simulink model "AS_KPI"  (R2024b)
settings: Solver=VariableStepAuto  StartTime=0.0  StopTime=10.0  RelTol=1e-3
settings Model: Creator=wangjianhai  LastModifiedBy=wangjianhai
settings ConfigComp: CovBoundaryAbsTol=1.0e-5

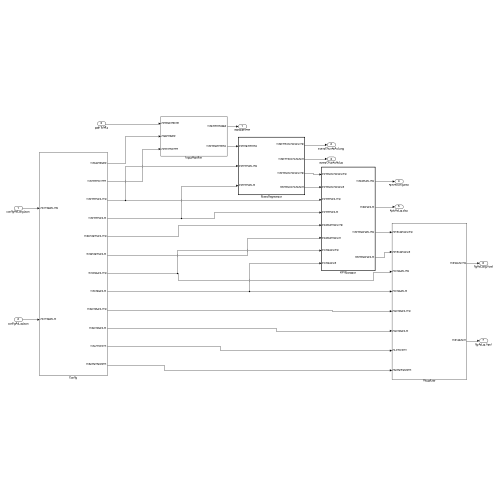
[thumbnail: Simulink's stored preview of the top-level diagram]
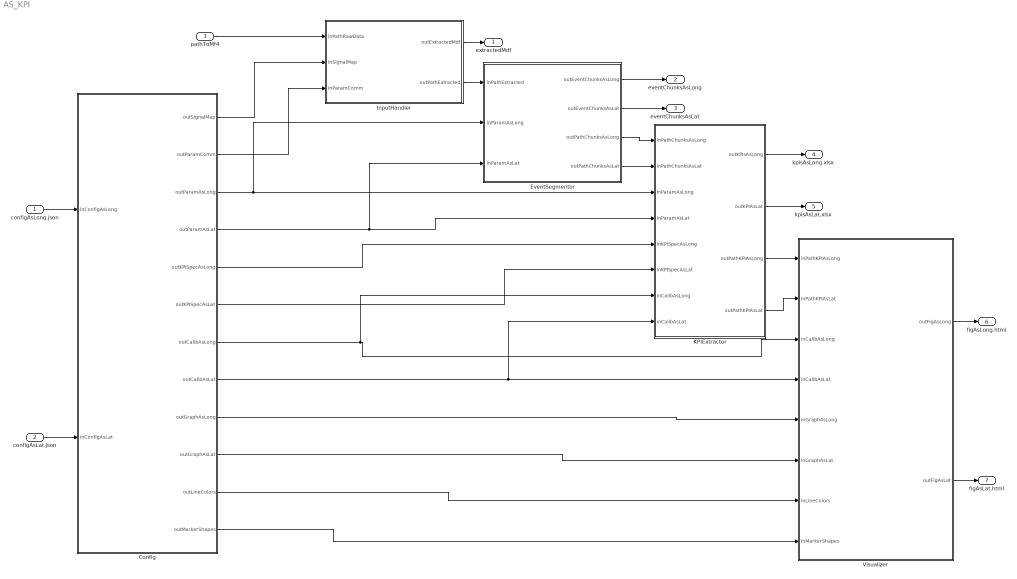
== system AS_KPI ==
  configAsLong.json : Inport
  configAsLat.json : Inport  Port=2
  pathToMf4 : Inport  Port=3
  Config : Subsystem
  EventSegmentor : Subsystem  TreatAsAtomicUnit=on
  InputHandler : Subsystem
  KPIExtractor : Subsystem  AutoFrameSizeCalculation=on
  Visualizer : Subsystem
  extractedMdf : Outport  VectorParamsAs1DForOutWhenUnconnected=off
  eventChunksAsLong : Outport  Port=2  VectorParamsAs1DForOutWhenUnconnected=off
  eventChunksAsLat : Outport  Port=3  VectorParamsAs1DForOutWhenUnconnected=off
  kpisAsLong.xlsx : Outport  Port=4  VectorParamsAs1DForOutWhenUnconnected=off
  kpisAsLat.xlsx : Outport  Port=5  VectorParamsAs1DForOutWhenUnconnected=off
  figAsLong.html : Outport  Port=6  VectorParamsAs1DForOutWhenUnconnected=off
  figAsLat.html : Outport  Port=7  VectorParamsAs1DForOutWhenUnconnected=off
  wires:
  Visualizer/2(outFigAsLat) -> figAsLat.html/1
  KPIExtractor/4(outPathKPIAsLat) -> Visualizer/2(inPathKPIAsLat)
  KPIExtractor/2(outKPIAsLat) -> kpisAsLat.xlsx/1
  KPIExtractor/1(outKPIsAsLong) -> kpisAsLong.xlsx/1
  InputHandler/2(outPathExtracted) -> EventSegmentor/1(inPathExtracted)
  Config/1(outSignalMap) -> InputHandler/2(inSignalMap)
  Config/11(outLineColors) -> Visualizer/7(inLineColors)
  Config/9(outGraphAsLong) -> Visualizer/5(inGraphAsLong)
  Config/10(outGraphAsLat) -> Visualizer/6(inGraphAsLat)
  EventSegmentor/3(outPathChunksAsLong) -> KPIExtractor/1(inPathChunksAsLong)
  Visualizer/1(outFigAsLong) -> figAsLong.html/1
  Config/7(outCalibAsLong) -> KPIExtractor/7(inCalibAsLong), Visualizer/3(inCalibAsLong)
  KPIExtractor/3(outPathKPIAsLong) -> Visualizer/1(inPathKPIAsLong)
  EventSegmentor/1(outEventChunksAsLong) -> eventChunksAsLong/1
  InputHandler/1(outExtractedMdf) -> extractedMdf/1
  Config/5(outKPISpecAsLong) -> KPIExtractor/5(inKPISpecAsLong)
  Config/4(outParamAsLat) -> EventSegmentor/3(inParamAsLat), KPIExtractor/4(inParamAsLat)
  Config/3(outParamAsLong) -> EventSegmentor/2(inParamAsLong), KPIExtractor/3(inParamAsLong)
  Config/12(outMarkerShapes) -> Visualizer/8(inMarkerShapes)
  Config/2(outParamComm) -> InputHandler/3(inParamComm)
  EventSegmentor/4(outPathChunksAsLat) -> KPIExtractor/2(inPathChunksAsLat)
  Config/8(outCalibAsLat) -> Visualizer/4(inCalibAsLat), KPIExtractor/8(inCalibAsLat)
  pathToMf4/1 -> InputHandler/1(inPathRawData)
  EventSegmentor/2(outEventChunksAsLat) -> eventChunksAsLat/1
  Config/6(outKPISpecAsLat) -> KPIExtractor/6(inKPISpecAsLat)
  configAsLat.json/1 -> Config/2(inConfigAsLat)
  configAsLong.json/1 -> Config/1(inConfigAsLong)

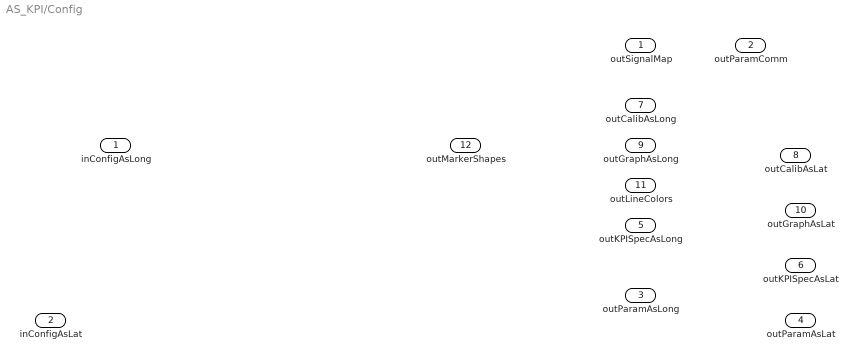
== system AS_KPI/Config ==
  inConfigAsLong : Inport
  inConfigAsLat : Inport  Port=2
  outSignalMap : Outport
  outParamComm : Outport  Port=2
  outParamAsLong : Outport  Port=3
  outParamAsLat : Outport  Port=4
  outKPISpecAsLong : Outport  Port=5
  outKPISpecAsLat : Outport  Port=6
  outCalibAsLong : Outport  Port=7
  outCalibAsLat : Outport  Port=8
  outGraphAsLong : Outport  Port=9
  outGraphAsLat : Outport  Port=10
  outLineColors : Outport  Port=11
  outMarkerShapes : Outport  Port=12

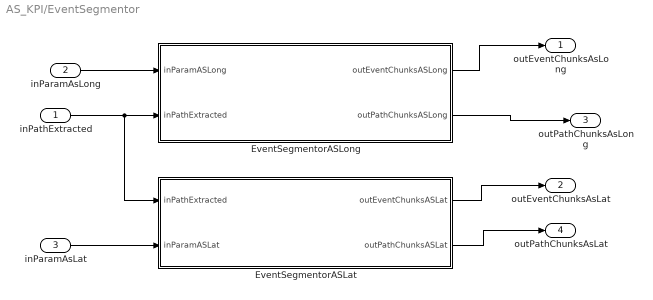
== system AS_KPI/EventSegmentor ==
  inPathExtracted : Inport
  inParamAsLong : Inport  Port=2
  inParamAsLat : Inport  Port=3
  EventSegmentorASLat : Subsystem  TreatAsAtomicUnit=on
  EventSegmentorASLong : Subsystem  TreatAsAtomicUnit=on
  outEventChunksAsLong : Outport
  outEventChunksAsLat : Outport  Port=2
  outPathChunksAsLong : Outport  Port=3
  outPathChunksAsLat : Outport  Port=4
  wires:
  inPathExtracted/1 -> EventSegmentorASLat/1(inPathExtracted), EventSegmentorASLong/2(inPathExtracted)
  inParamAsLong/1 -> EventSegmentorASLong/1(inParamASLong)
  inParamAsLat/1 -> EventSegmentorASLat/2(inParamASLat)
  EventSegmentorASLong/1(outEventChunksASLong) -> outEventChunksAsLong/1
  EventSegmentorASLong/2(outPathChunksASLong) -> outPathChunksAsLong/1
  EventSegmentorASLat/1(outEventChunksASLat) -> outEventChunksAsLat/1
  EventSegmentorASLat/2(outPathChunksASLat) -> outPathChunksAsLat/1

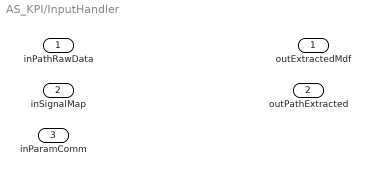
== system AS_KPI/InputHandler ==
  inPathRawData : Inport
  inSignalMap : Inport  Port=2
  inParamComm : Inport  Port=3
  outExtractedMdf : Outport
  outPathExtracted : Outport  Port=2

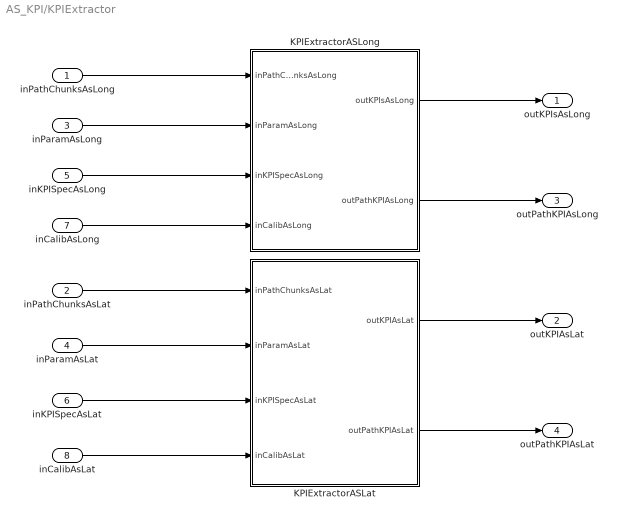
== system AS_KPI/KPIExtractor ==
  inPathChunksAsLong : Inport
  inPathChunksAsLat : Inport  Port=2
  inParamAsLong : Inport  Port=3
  inParamAsLat : Inport  Port=4
  inKPISpecAsLong : Inport  Port=5
  inKPISpecAsLat : Inport  Port=6
  inCalibAsLong : Inport  Port=7
  inCalibAsLat : Inport  Port=8
  KPIExtractorASLat : Subsystem  AutoFrameSizeCalculation=on
  KPIExtractorASLong : Subsystem  AutoFrameSizeCalculation=on
  outKPIsAsLong : Outport  VectorParamsAs1DForOutWhenUnconnected=off
  outKPIAsLat : Outport  Port=2  VectorParamsAs1DForOutWhenUnconnected=off
  outPathKPIAsLong : Outport  Port=3  VectorParamsAs1DForOutWhenUnconnected=off
  outPathKPIAsLat : Outport  Port=4  VectorParamsAs1DForOutWhenUnconnected=off
  wires:
  KPIExtractorASLong/1(outKPIsAsLong) -> outKPIsAsLong/1
  KPIExtractorASLat/1(outKPIAsLat) -> outKPIAsLat/1
  KPIExtractorASLong/2(outPathKPIAsLong) -> outPathKPIAsLong/1
  KPIExtractorASLat/2(outPathKPIAsLat) -> outPathKPIAsLat/1
  inCalibAsLong/1 -> KPIExtractorASLong/4(inCalibAsLong)
  inParamAsLong/1 -> KPIExtractorASLong/2(inParamAsLong)
  inPathChunksAsLong/1 -> KPIExtractorASLong/1(inPathChunksAsLong)
  inKPISpecAsLong/1 -> KPIExtractorASLong/3(inKPISpecAsLong)
  inParamAsLat/1 -> KPIExtractorASLat/2(inParamAsLat)
  inPathChunksAsLat/1 -> KPIExtractorASLat/1(inPathChunksAsLat)
  inKPISpecAsLat/1 -> KPIExtractorASLat/3(inKPISpecAsLat)
  inCalibAsLat/1 -> KPIExtractorASLat/4(inCalibAsLat)

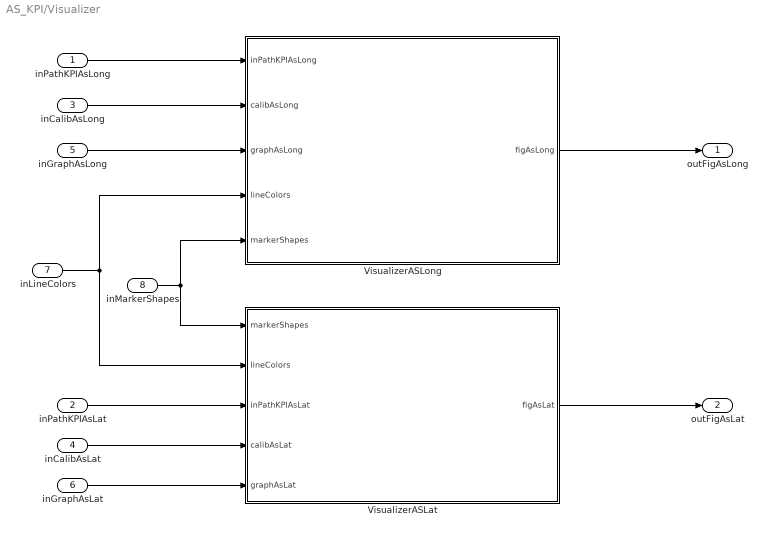
== system AS_KPI/Visualizer ==
  inPathKPIAsLong : Inport
  inPathKPIAsLat : Inport  Port=2
  inCalibAsLong : Inport  Port=3
  inCalibAsLat : Inport  Port=4
  inGraphAsLong : Inport  Port=5
  inGraphAsLat : Inport  Port=6
  inLineColors : Inport  Port=7
  inMarkerShapes : Inport  Port=8
  VisualizerASLat : Subsystem
  VisualizerASLong : Subsystem
  outFigAsLong : Outport
  outFigAsLat : Outport  Port=2
  wires:
  inGraphAsLong/1 -> VisualizerASLong/3(graphAsLong)
  inCalibAsLong/1 -> VisualizerASLong/2(calibAsLong)
  inPathKPIAsLong/1 -> VisualizerASLong/1(inPathKPIAsLong)
  inCalibAsLat/1 -> VisualizerASLat/4(calibAsLat)
  inGraphAsLat/1 -> VisualizerASLat/5(graphAsLat)
  inMarkerShapes/1 -> VisualizerASLat/1(markerShapes), VisualizerASLong/5(markerShapes)
  inLineColors/1 -> VisualizerASLat/2(lineColors), VisualizerASLong/4(lineColors)
  inPathKPIAsLat/1 -> VisualizerASLat/3(inPathKPIAsLat)
  VisualizerASLat/1(figAsLat) -> outFigAsLat/1
  VisualizerASLong/1(figAsLong) -> outFigAsLong/1

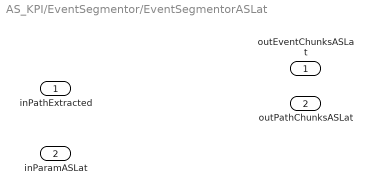
== system AS_KPI/EventSegmentor/EventSegmentorASLat ==
  inPathExtracted : Inport
  inParamASLat : Inport  Port=2
  outEventChunksASLat : Outport
  outPathChunksASLat : Outport  Port=2

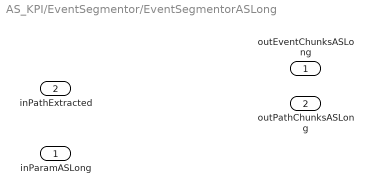
== system AS_KPI/EventSegmentor/EventSegmentorASLong ==
  inParamASLong : Inport
  inPathExtracted : Inport  Port=2
  outEventChunksASLong : Outport
  outPathChunksASLong : Outport  Port=2

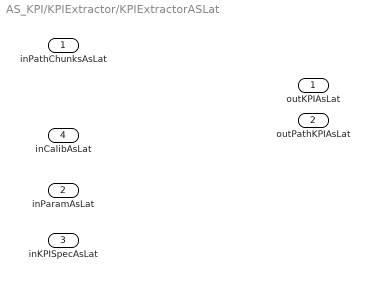
== system AS_KPI/KPIExtractor/KPIExtractorASLat ==
  inPathChunksAsLat : Inport
  inParamAsLat : Inport  Port=2
  inKPISpecAsLat : Inport  Port=3
  inCalibAsLat : Inport  Port=4
  outKPIAsLat : Outport  VectorParamsAs1DForOutWhenUnconnected=off
  outPathKPIAsLat : Outport  Port=2  VectorParamsAs1DForOutWhenUnconnected=off

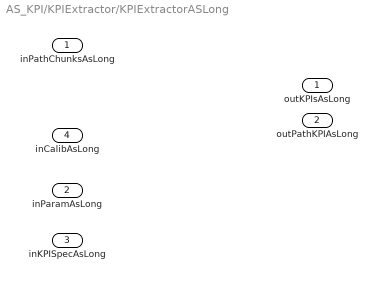
== system AS_KPI/KPIExtractor/KPIExtractorASLong ==
  inPathChunksAsLong : Inport
  inParamAsLong : Inport  Port=2
  inKPISpecAsLong : Inport  Port=3
  inCalibAsLong : Inport  Port=4
  outKPIsAsLong : Outport  VectorParamsAs1DForOutWhenUnconnected=off
  outPathKPIAsLong : Outport  Port=2  VectorParamsAs1DForOutWhenUnconnected=off

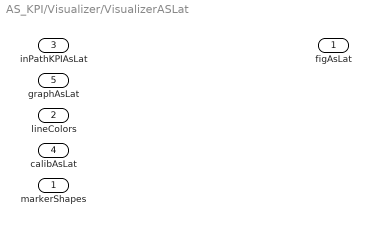
== system AS_KPI/Visualizer/VisualizerASLat ==
  markerShapes : Inport
  lineColors : Inport  Port=2
  inPathKPIAsLat : Inport  Port=3
  calibAsLat : Inport  Port=4
  graphAsLat : Inport  Port=5
  figAsLat : Outport

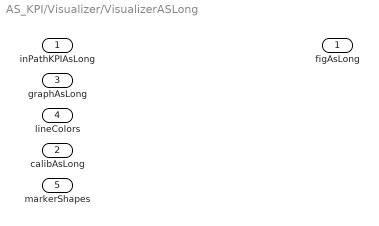
== system AS_KPI/Visualizer/VisualizerASLong ==
  inPathKPIAsLong : Inport
  calibAsLong : Inport  Port=2
  graphAsLong : Inport  Port=3
  lineColors : Inport  Port=4
  markerShapes : Inport  Port=5
  figAsLong : Outport
